simulink model "EngineState_harness"  (Simulink 7.7)
settings: Solver=FixedStepDiscrete  SolverMode=SingleTasking  StartTime=0.0  StopTime=100  FixedStep=0.01  RelTol=1e-3
InitFcn:
  | if signalbuilder('EngineState_harness/Signal_Builder','activegroup') == 11
  |   CD_PANEL_SHUTDOWN_FUNCTION.DataType = 'uint8';
  |   CD_PANEL_SHUTDOWN_FUNCTION.Value = 255;
  | else
  |   CD_PANEL_SHUTDOWN_FUNCTION.DataType = 'uint8';
  |   CD_PANEL_SHUTDOWN_FUNCTION.Value = 0;
  | end
  | 
  | if signalbuilder('EngineState_harness/Signal_Builder','activegroup') == 2
  |   CD_ECU_FUNCTION.DataType = 'uint8';
  |   CD_ECU_FUNCTION.Value = 0;
  | elseif signalbuilder('EngineState_harness/Signal_Builder','activegroup') == 15
  |   CD_ECU_FUNCTION.DataType = 'uint8';
  |   CD_ECU_FUNCTION.Value = 0;
  | else
  |   CD_ECU_FUNCTION.DataType = 'uint8';
  |   CD_ECU_FUNCTION.Value = 255;
  | end
undefined symbols (not defined in the file): sigbuilder_block, srate
CloseFcn:
  | rtwprivate ssgencode ModelCloseRequest sle_main_controller
settings Model: Creator=smindema  LastModifiedBy=aliebel  CovMetricSettings=dcmw  CovHTMLOptions=-aTS=1 -bRG=1 -bTC=1 -hTR=0 -nFC=0 -scm=1 -bcm=1 -xEv=0  covSaveCumulativeToWorkspaceVar=off  CovSaveSingleToWorkspaceVar=off  CovModelRefEnable=off
settings MATStruct: SampleTime=0.01  Offset=0  Priority=[1.0]
settings DataIOCC: LimitDataPoints=off  SaveOutput=off  SaveTime=off
settings OptimizationCC: BlockReduction=off  InlineParams=on  ExpressionFolding=off  StateBitsets=on  DataBitsets=on  UseTempVars=on  InitFltsAndDblsToZero=on  NoFixptDivByZeroProtection=on  EfficientFloat2IntCast=on  OptimizeModelRefInitCode=on
settings DebuggingCC: SaveWithParameterizedLinksMsg=none  MultiTaskDSMMsg=warning  MultiTaskCondExecSysMsg=none  IntegerOverflowMsg=none  ModelReferenceCSMismatchMessage=warning
settings HardwareCC: ProdBitPerInt=16  ProdBitPerPointer=16  ProdIntDivRoundTo=Zero  ProdEndianess=BigEndian  ProdWordSize=16  ProdHWDeviceType=Motorola HC12
settings ModelReferenceCC: ModelReferenceNumInstancesAllowed=Single
settings SFSimCC: SimCustomHeaderCode="#include \"SendMsgNow.h\""  SimUserSources=SendMsgNow_Blank.c  SimUserIncludeDirs=functions
settings RTWCC: SystemTargetFile=ert.tlc  GenCodeOnly=on  TemplateMakefile=ert_default_tmf  Description=Real-Time Workshop Embedded Coder (no auto configuration)  GenerateReport=on  RetainRTWFile=on  ProcessScript=ert_make_rtw_hook  IncludeHyperlinkInReport=on  LaunchReport=on  IncludeERTFirstTime=on
settings RTWCC: CustomHeaderCode=|
  | #include "cpp_req_defines.h"
  | #include "hw_fin.h"
  | #include "cdata.h"
settings CodeAppCC: IgnoreCustomStorageClasses=off  DefineNamingRule=UpperCase
settings ERTTargetCC: TargetFcnLib=ansi_tfl_tmw.mat  FunctionExecutionProfile=off  MultiwordLength=2048  GenerateSampleERTMain=on  IncludeMdlTerminateFcn=off  SuppressErrorStatus=on  SupportAbsoluteTime=off  SupportNonFinite=off  SupportComplex=off  PurelyIntegerCode=on  ERTCustomFileTemplate=gen_rtw_req_defines_h.tlc  GlobalDataDefinition=InSeparateSourceFile  GlobalDataReference=InSeparateHeaderFile  ConvertIfToSwitch=off

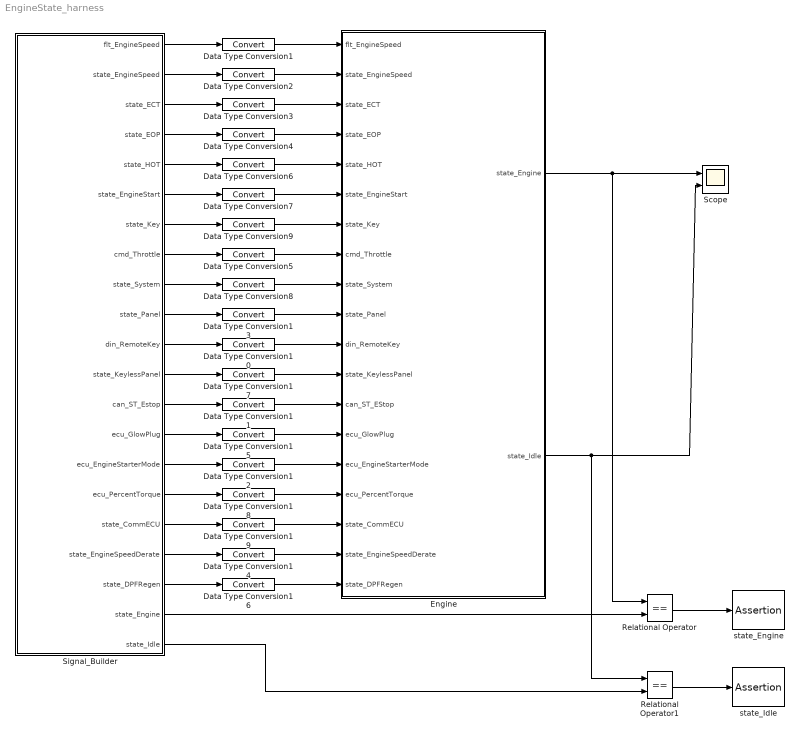
== system EngineState_harness ==
  Data Type Conversion{1..19} (19 alike) : DataTypeConversion
  Engine : Subsystem  TreatAsAtomicUnit=on  SystemSampleTime=srate  RTWFileName=mod_System
      settings: RTWSystemCode=Function  RTWFcnNameOpts=Use subsystem name  RTWFileNameOpts=User specified
  Relational Operator : RelationalOperator  Operator===  OutDataTypeStr=boolean
  Relational Operator1 : RelationalOperator  Operator===  OutDataTypeStr=boolean
  Scope : Scope  NumInputPorts=2
      settings: TimeRange=100  YMin=0~-5  YMax=5~5  MaxDataPoints=50000
  Signal_Builder : Subsystem  Tag=STV Subsys  LoadFcn=sigbuilder_block('load',[1440 133.5 1440 753 ]);  StartFcn=sigbuilder_block('start');  StopFcn=sigbuilder_block('stop');  ClipboardFcn=sigbuilder_block('clipboard');  mask(Sigbuilder block){}
      mask help: Sigbuilder GUI
      mask init:
      | if ~strcmp(get_param(bdroot(gcbh),'SimulationStatus'),'stopped') tuvar = sigbuilder_block('maskInit'); end
      settings: CopyFcn=sigbuilder_block('copy');  DeleteFcn=sigbuilder_block('delete');  ModelCloseFcn=sigbuilder_block('modelClose');  PreSaveFcn=sigbuilder_block('preSave');  NameChangeFcn=sigbuilder_block('namechange');  OpenFcn=sigbuilder_block('open',[1440 133.5 1440 753 ]);  CloseFcn=sigbuilder_block('close');
      mask Display: plot(0,0,100,100,[10,10,40,40,10],[80,20,20,80,80],[40,10],[50,50], [40,27,10],[65,72,56],[40,25,25,10],[28,28,43,43]);
  state_Engine : Assertion  Enabled=off
  state_Idle : Assertion  Enabled=off
  wires:
  Signal_Builder/1(flt_EngineSpeed) -> Data Type Conversion1/1
  Signal_Builder/2(state_EngineSpeed) -> Data Type Conversion2/1
  Signal_Builder/3(state_ECT) -> Data Type Conversion3/1
  Signal_Builder/4(state_EOP) -> Data Type Conversion4/1
  Signal_Builder/5(state_HOT) -> Data Type Conversion6/1
  Signal_Builder/6(state_EngineStart) -> Data Type Conversion7/1
  Signal_Builder/7(state_Key) -> Data Type Conversion9/1
  Engine/1(state_Engine) -> Relational Operator/1, Scope/1
  Relational Operator/1 -> state_Engine/1
  Signal_Builder/20(state_Engine) -> Relational Operator/2
  Data Type Conversion1/1 -> Engine/1(flt_EngineSpeed)
  Data Type Conversion2/1 -> Engine/2(state_EngineSpeed)
  Data Type Conversion3/1 -> Engine/3(state_ECT)
  Data Type Conversion4/1 -> Engine/4(state_EOP)
  Data Type Conversion6/1 -> Engine/5(state_HOT)
  Data Type Conversion7/1 -> Engine/6(state_EngineStart)
  Data Type Conversion9/1 -> Engine/7(state_Key)
  Signal_Builder/9(state_System) -> Data Type Conversion8/1
  Signal_Builder/10(state_Panel) -> Data Type Conversion13/1
  Signal_Builder/14(ecu_GlowPlug) -> Data Type Conversion15/1
  Signal_Builder/12(state_KeylessPanel) -> Data Type Conversion17/1
  Signal_Builder/16(ecu_PercentTorque) -> Data Type Conversion18/1
  Signal_Builder/17(state_CommECU) -> Data Type Conversion19/1
  Data Type Conversion8/1 -> Engine/9(state_System)
  Data Type Conversion13/1 -> Engine/10(state_Panel)
  Data Type Conversion15/1 -> Engine/14(ecu_GlowPlug)
  Data Type Conversion17/1 -> Engine/12(state_KeylessPanel)
  Data Type Conversion18/1 -> Engine/16(ecu_PercentTorque)
  Data Type Conversion19/1 -> Engine/17(state_CommECU)
  Signal_Builder/8(cmd_Throttle) -> Data Type Conversion5/1
  Signal_Builder/11(din_RemoteKey) -> Data Type Conversion10/1
  Signal_Builder/13(can_ST_Estop) -> Data Type Conversion11/1
  Signal_Builder/15(ecu_EngineStarterMode) -> Data Type Conversion12/1
  Data Type Conversion12/1 -> Engine/15(ecu_EngineStarterMode)
  Data Type Conversion11/1 -> Engine/13(can_ST_EStop)
  Data Type Conversion10/1 -> Engine/11(din_RemoteKey)
  Data Type Conversion5/1 -> Engine/8(cmd_Throttle)
  Signal_Builder/18(state_EngineSpeedDerate) -> Data Type Conversion14/1
  Signal_Builder/19(state_DPFRegen) -> Data Type Conversion16/1
  Data Type Conversion14/1 -> Engine/18(state_EngineSpeedDerate)
  Data Type Conversion16/1 -> Engine/19(state_DPFRegen)
  Relational Operator1/1 -> state_Idle/1
  Signal_Builder/21(state_Idle) -> Relational Operator1/2
  Engine/2(state_Idle) -> Relational Operator1/1, Scope/2

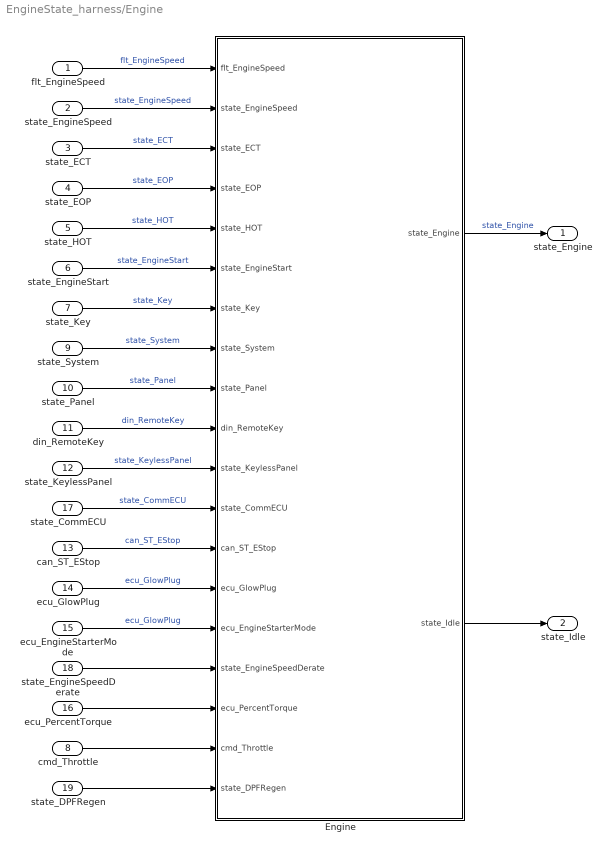
== system EngineState_harness/Engine ==
  flt_EngineSpeed : Inport
  state_EngineSpeed : Inport  Port=2  OutDataTypeStr=uint8
  state_ECT : Inport  Port=3  OutDataTypeStr=uint8
  state_EOP : Inport  Port=4  OutDataTypeStr=uint8
  state_HOT : Inport  Port=5  OutDataTypeStr=uint8
  state_EngineStart : Inport  Port=6  OutDataTypeStr=uint8
  state_Key : Inport  Port=7  OutDataTypeStr=uint8
  cmd_Throttle : Inport  Port=8
  state_System : Inport  Port=9  OutDataTypeStr=uint8
  state_Panel : Inport  Port=10  OutDataTypeStr=uint8
  din_RemoteKey : Inport  Port=11  OutDataTypeStr=uint8
  state_KeylessPanel : Inport  Port=12  OutDataTypeStr=uint8
  can_ST_EStop : Inport  Port=13  OutDataTypeStr=uint8
  ecu_GlowPlug : Inport  Port=14  OutDataTypeStr=uint8
  ecu_EngineStarterMode : Inport  Port=15  OutDataTypeStr=uint8
  ecu_PercentTorque : Inport  Port=16
  state_CommECU : Inport  Port=17  OutDataTypeStr=uint8
  state_EngineSpeedDerate : Inport  Port=18  OutDataTypeStr=uint8
  state_DPFRegen : Inport  Port=19
  Engine : Stateflow chart  TreatAsAtomicUnit=on
  state_Engine : Outport  OutDataTypeStr=uint8
  state_Idle : Outport  Port=2  OutDataTypeStr=uint8
  wires:
  Engine/1(state_Engine) -> state_Engine/1  "state_Engine"
  flt_EngineSpeed/1 -> Engine/1(flt_EngineSpeed)  "flt_EngineSpeed"
  state_EngineSpeed/1 -> Engine/2(state_EngineSpeed)  "state_EngineSpeed"
  state_ECT/1 -> Engine/3(state_ECT)  "state_ECT"
  state_EOP/1 -> Engine/4(state_EOP)  "state_EOP"
  state_HOT/1 -> Engine/5(state_HOT)  "state_HOT"
  state_EngineStart/1 -> Engine/6(state_EngineStart)  "state_EngineStart"
  state_Key/1 -> Engine/7(state_Key)  "state_Key"
  state_System/1 -> Engine/8(state_System)  "state_System"
  state_Panel/1 -> Engine/9(state_Panel)  "state_Panel"
  din_RemoteKey/1 -> Engine/10(din_RemoteKey)  "din_RemoteKey"
  state_KeylessPanel/1 -> Engine/11(state_KeylessPanel)  "state_KeylessPanel"
  state_CommECU/1 -> Engine/12(state_CommECU)  "state_CommECU"
  can_ST_EStop/1 -> Engine/13(can_ST_EStop)  "can_ST_EStop"
  Engine/2(state_Idle) -> state_Idle/1
  ecu_GlowPlug/1 -> Engine/14(ecu_GlowPlug)  "ecu_GlowPlug"
  ecu_EngineStarterMode/1 -> Engine/15(ecu_EngineStarterMode)  "ecu_GlowPlug"
  state_EngineSpeedDerate/1 -> Engine/16(state_EngineSpeedDerate)
  ecu_PercentTorque/1 -> Engine/17(ecu_PercentTorque)
  cmd_Throttle/1 -> Engine/18(cmd_Throttle)
  state_DPFRegen/1 -> Engine/19(state_DPFRegen)

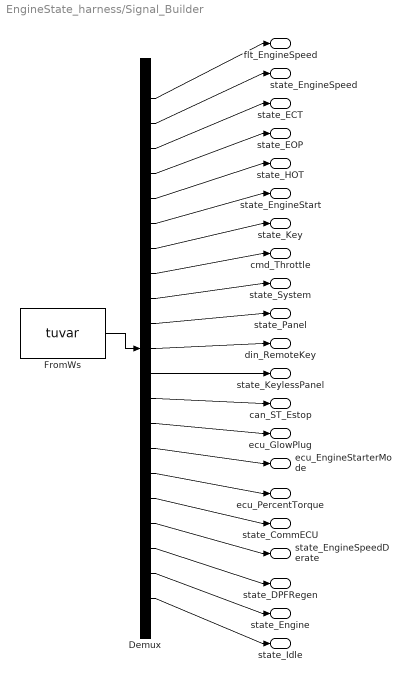
== system EngineState_harness/Signal_Builder ==
  Demux : Demux  Tag=STV Demux  Outputs=21
  FromWs : FromWorkspace  Tag=STV FromWs  VariableName=tuvar  SampleTime=0  SigBuilderData=DataTag0  VnvData=DataTag1
  flt_EngineSpeed : Outport  Tag=STV Outport
  state_EngineSpeed : Outport  Tag=STV Outport  Port=2
  state_ECT : Outport  Tag=STV Outport  Port=3
  state_EOP : Outport  Tag=STV Outport  Port=4
  state_HOT : Outport  Tag=STV Outport  Port=5
  state_EngineStart : Outport  Tag=STV Outport  Port=6
  state_Key : Outport  Tag=STV Outport  Port=7
  cmd_Throttle : Outport  Tag=STV Outport  Port=8
  state_System : Outport  Tag=STV Outport  Port=9
  state_Panel : Outport  Tag=STV Outport  Port=10
  din_RemoteKey : Outport  Tag=STV Outport  Port=11
  state_KeylessPanel : Outport  Tag=STV Outport  Port=12
  can_ST_Estop : Outport  Tag=STV Outport  Port=13
  ecu_GlowPlug : Outport  Tag=STV Outport  Port=14
  ecu_EngineStarterMode : Outport  Tag=STV Outport  Port=15
  ecu_PercentTorque : Outport  Tag=STV Outport  Port=16
  state_CommECU : Outport  Tag=STV Outport  Port=17
  state_EngineSpeedDerate : Outport  Tag=STV Outport  Port=18
  state_DPFRegen : Outport  Tag=STV Outport  Port=19
  state_Engine : Outport  Tag=STV Outport  Port=20
  state_Idle : Outport  Tag=STV Outport  Port=21
  wires:
  FromWs/1 -> Demux/1
  Demux/1 -> flt_EngineSpeed/1
  Demux/2 -> state_EngineSpeed/1
  Demux/3 -> state_ECT/1
  Demux/4 -> state_EOP/1
  Demux/5 -> state_HOT/1
  Demux/6 -> state_EngineStart/1
  Demux/7 -> state_Key/1
  Demux/8 -> cmd_Throttle/1
  Demux/9 -> state_System/1
  Demux/10 -> state_Panel/1
  Demux/11 -> din_RemoteKey/1
  Demux/12 -> state_KeylessPanel/1
  Demux/13 -> can_ST_Estop/1
  Demux/14 -> ecu_GlowPlug/1
  Demux/15 -> ecu_EngineStarterMode/1
  Demux/16 -> ecu_PercentTorque/1
  Demux/17 -> state_CommECU/1
  Demux/18 -> state_EngineSpeedDerate/1
  Demux/19 -> state_DPFRegen/1
  Demux/20 -> state_Engine/1
  Demux/21 -> state_Idle/1

== stateflow chart Engine/Engine ==
  state SHUTDOWN
    en:state_Engine = SHUTDOWN;
    en:SendMsg_03_Now();
    (junction 14) -> (junction 17) [order 2]
    SHUTDOWN -> (junction 14)
    (junction 14) -> (junction 15) [order 1] : [(CD_ECU_FUNCTION != NON_FUNCTIONAL)...
        | && (flt_EngineSpeed > CD_ENGINE_SPEED_NOT_RUNNING)]
    (junction 15) -> (junction 16) : {
        | SendMsg_ShutdownEngine_Now();
        | }
    (junction 16) -> (junction 17)
  state ST_SHUTDOWN
    en:state_Engine = ENGINE_OFF;
    en:SendMsg_03_Now();
    (junction 22) -> (junction 24) [order 2]
    (junction 22) -> (junction 23) [order 1] : [(CD_ECU_FUNCTION != NON_FUNCTIONAL)...
        | && (flt_EngineSpeed > CD_ENGINE_SPEED_NOT_RUNNING)]
    (junction 25) -> (junction 24)
    (junction 23) -> (junction 25) : {
        | SendMsg_ShutdownEngine_Now();
        | }
    ST_SHUTDOWN -> (junction 22) [order 1]
  state NORMAL
    state NOT_RUNNING
      state WAIT_TO_START
        en:state_Engine = ENGINE_INITIALIZE;
        en:debounceCount = 0;
        du:debounceCount++;
      state NOT_RUNNING
        en:state_Engine = ENGINE_NOT_RUNNING;
        en:SendMsg_03_Now();
      WAIT_TO_START -> NORMAL.NOT_RUNNING.NOT_RUNNING : [((debounceCount >= CD_ECU_DEBOUNCE_WAIT_TO_START) && (ecu_GlowPlug != ACTIVE) && (state_CommECU == NORMAL))...
          | || (CD_ECU_FUNCTION == NON_FUNCTIONAL)]
      (default) -> NORMAL.NOT_RUNNING.NOT_RUNNING
    state CRANKING
      en:state_Engine = ENGINE_CRANKING;
      en:SendMsg_03_Now();
    state RUNNING
      en:state_Engine = ENGINE_RUNNING;
      en:SendMsg_03_Now();
      ex:state_Idle = INACTIVE;
      state COUNT_IDLE
        en:state_Idle = ACTIVE;
      state NOT_IDLE
        en:state_Idle = INACTIVE;
        en:idle_Speed = flt_EngineSpeed;
        en:debounceIdle = 0;
        note: If engine speed changes by x amount reset counter, other wise if it remains with
            | in the window, increment counter.
        NOT_IDLE -> (junction 18) [order 1]
        (junction 18) -> (junction 19) [order 1] : [(CD_IDLE_TIME_FUNCTION != NON_FUNCTIONAL)...
            | && (flt_EngineSpeed <= idle_Speed + CD_IDLE_ENGINE_SPEED_OFFSET)...
            | && (flt_EngineSpeed >= idle_Speed - CD_IDLE_ENGINE_SPEED_OFFSET)...
            | && (ecu_PercentTorque <= CD_IDLE_TORQUE_LEVEL)]
        (junction 18) -> (junction 20) [order 2] : {
            | idle_Speed = flt_EngineSpeed;
            | debounceIdle = 0;
            | }
        (junction 19) -> (junction 21) : {
            | debounceIdle++;
            | }
        (junction 21) -> (junction 20)
      (default) -> NOT_IDLE
      NOT_IDLE -> COUNT_IDLE [order 1] : [(debounceIdle >= CD_IDLE_DEBOUNCE_ACTIVE)...
          | || (cmd_Throttle == CD_LOW_IDLE_COMMAND)]
      COUNT_IDLE -> NOT_IDLE : [((flt_EngineSpeed >= idle_Speed + CD_IDLE_ENGINE_SPEED_OFFSET)...
          |    || (flt_EngineSpeed <= idle_Speed - CD_IDLE_ENGINE_SPEED_OFFSET)...
          |    || (ecu_PercentTorque > CD_IDLE_TORQUE_LEVEL))...
          | &&  (cmd_Throttle != CD_LOW_IDLE_COMMAND)]
    NORMAL.NOT_RUNNING -> CRANKING [order 1] : [((state_EngineStart == ACTIVE))...
        | && (state_Key == ACTIVE)...
        | && (state_System == SYS_NORMAL)...
        | && (((state_CommECU != NO_COMMUNICATION) && (ecu_EngineStarterMode != STARTER_INHIBITED)) || (CD_ECU_FUNCTION == NON_FUNCTIONAL))]
    CRANKING -> RUNNING [order 1] : [(flt_EngineSpeed >= CD_ENGINE_SPEED_RUNNING)]
    NORMAL.NOT_RUNNING -> RUNNING [order 2] : [(flt_EngineSpeed >= CD_ENGINE_SPEED_RUNNING)...
        | && (state_System == SYS_NORMAL)]
    RUNNING -> NORMAL.NOT_RUNNING [order 2] : [((flt_EngineSpeed <= CD_ENGINE_SPEED_NOT_RUNNING)...
        | || (state_System != SYS_NORMAL))]
    CRANKING -> NORMAL.NOT_RUNNING [order 2] : [((state_EngineStart != ACTIVE))...
        | || (state_Key != ACTIVE)...
        | || (state_System != SYS_NORMAL)...
        | || (ecu_EngineStarterMode == STARTER_INHIBITED)]
    (default) -> WAIT_TO_START
  RUNNING -> SHUTDOWN [order 1] : [(state_ECT == SHUTDOWN)...
      | || (state_EOP == SHUTDOWN)...
      | || (state_HOT == SHUTDOWN)...
      | || (state_EngineSpeed == SHUTDOWN)...
      | || (state_KeylessPanel == NO_COMMUNICATION)...
      | || (((state_CommECU == NO_COMMUNICATION) || (state_EngineSpeedDerate == SHUTDOWN)) && (CD_ECU_FUNCTION != NON_FUNCTIONAL))...
      | || ((state_Panel == NO_COMMUNICATION) && (CD_PANEL_SHUTDOWN_FUNCTION != NON_FUNCTIONAL) && (din_RemoteKey != ACTIVE))...
      | || (state_DPFRegen == SHUTDOWN)]
  NORMAL -> SHUTDOWN [order 2] : [(state_Key == MULTIPLE)]
  NORMAL -> ST_SHUTDOWN [order 1] : [(can_ST_EStop == ACTIVE)]
  ST_SHUTDOWN -> NORMAL [order 1] : [(can_ST_EStop == INACTIVE)]
  (default) -> NORMAL
  data: state_Engine output uint8; flt_EngineSpeed input uint16; state_EngineSpeed input uint8; state_ECT input uint8; state_EOP input uint8; state_HOT input uint8; state_EngineStart input uint8; CD_ENGINE_SPEED_RUNNING parameter uint16; CD_ENGINE_SPEED_NOT_RUNNING parameter uint16; state_Key input uint8; ACTIVE parameter uint8 =1; ENGINE_CRANKING parameter uint8 =2; ENGINE_NOT_RUNNING parameter uint8 =1; ENGINE_RUNNING parameter uint8 =3; INACTIVE parameter uint8 =0; SHUTDOWN parameter uint8 =15; state_System input uint8; state_Panel input uint8; SYS_NORMAL parameter uint8; NO_COMMUNICATION parameter uint8; CD_PANEL_SHUTDOWN_FUNCTION parameter uint8; NON_FUNCTIONAL parameter uint8; MULTIPLE parameter uint8; ENGINE_OFF parameter uint8; din_RemoteKey input uint8; NORMAL parameter uint8; state_KeylessPanel input uint8; CD_ECU_FUNCTION parameter uint8; state_CommECU input uint8; can_ST_EStop input uint8; CD_IDLE_TIME_FUNCTION parameter uint8; CD_IDLE_DEBOUNCE_ACTIVE parameter uint16; CD_IDLE_ENGINE_SPEED_OFFSET parameter uint16; debounceIdle local uint16; state_Idle output uint8; ENGINE_INITIALIZE parameter uint8; CD_ECU_DEBOUNCE_WAIT_TO_START parameter uint16; ecu_GlowPlug input uint8; debounceCount local uint16; STARTER_INHIBITED parameter uint8; ecu_EngineStarterMode input uint8; state_EngineSpeedDerate input uint8; CD_IDLE_TORQUE_LEVEL parameter uint8; ecu_PercentTorque input int8; idle_Speed local uint16; cmd_Throttle input uint16; CD_LOW_IDLE_COMMAND parameter uint16; state_DPFRegen input uint8
